simulink model "ControlePD_5juntas"  (R2020a)
settings: Solver=FixedStepAuto  StartTime=0.0  StopTime=10  FixedStep=Ts
values from neighbouring files (symbols this model uses):
  Beff = 50    [controle.m]    (also in controle_FF.m; controle_PD.m)
  ganho_degrau = [0;0;0;0;0]    [controle.m]    (also in controle_PD.m)
  Jeff = 2.2    [controle.m]    (also in controle_FF.m = 0.5; controle_PD.m = 0.5)
  K = 17.7    [controle.m]    (also in controle_FF.m = 0.785398163397; controle_PD.m = 0.785398163397)
  Kd = (2*zeta*wn*Jeff - Beff)/K    (= -2.32768361582)    [controle.m]    (also in controle_FF.m = -44.5633840657; controle_PD.m = -44.5633840657)
  Kp = (wn^2*Jeff)/K    (= 0.497175141243)    [controle.m]    (also in controle_FF.m = 143.239448783; controle_PD.m = 143.239448783)
  N = 10    [controle.m]    (also in controle_FF.m = 3; controle_PD.m = 3)
  r = 1/100    (= 0.01)    [controle.m]    (also in controle_FF.m = 1./[231.22*4 139.138 139.138 231.22 231.22]; controle_PD.m = 1./[231.22*4 139.138 139.138 231.22 231.22])
  SP_theta = [0;0;0;0;0]    [controle.m]    (also in controle_FF.m = [0 0 0 0 0]; controle_PD.m)
  tempo_degrau = [0;0;0;0;0]    [controle.m]    (also in controle_PD.m)
libraries: simulink_extras x20
(part 3 of 3)

== matlab function ControlePD_5juntas/Perturbação/MATLAB Function ==
  data: M input; V input; tau1 output; G input; ddTh input
function tau1  = calcul_dk1(M, V, G, ddTh)

tau1 = M(1,2)*ddTh(2) + M(1,3)*ddTh(3) + M(1,4)*ddTh(4) + M(1,5)*ddTh(5) ...
       + V(1) + G(1);
